simulink subsystem "Linear2Global_AV"  (R2024b)
settings: Solver=VariableStepAuto  StartTime=0.0  StopTime=10.0  RelTol=1e-3
settings Model: Creator=marti  LastModifiedBy=marti

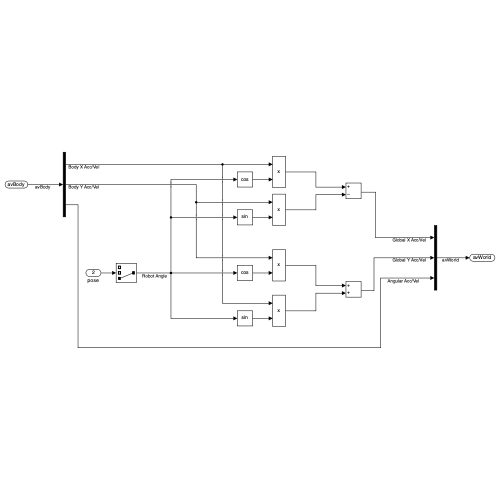
[thumbnail: Simulink's stored preview of the top-level diagram]
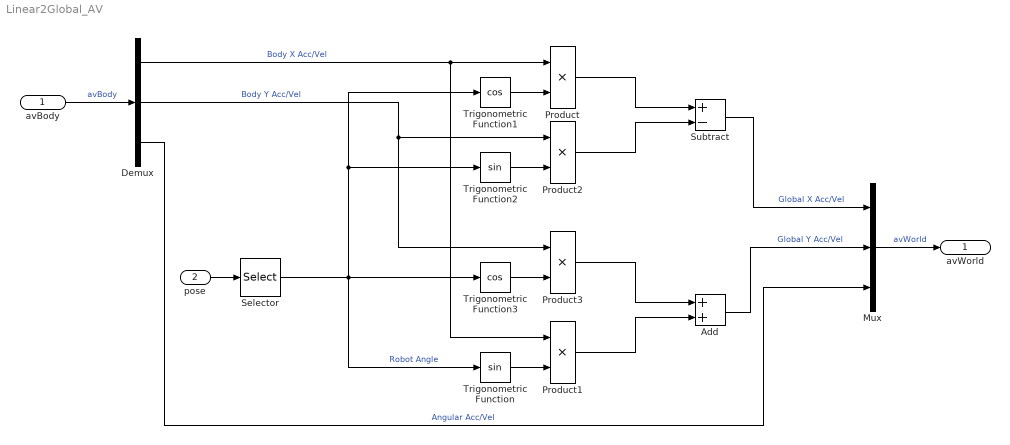
== system Linear2Global_AV ==
  avBody : Inport
  pose : Inport  Port=2
  Add : Sum
  Demux : Demux  Outputs=3
  Mux : Mux  Inputs=3
  Product{,1..3} (4 alike) : Product
  Selector : Selector  InputPortWidth=3  IndexOptions=Index vector (dialog)  Indices=3  OutputSizes=1
  Subtract : Sum  Inputs=+-
  Trigonometric Function : Trigonometry
  Trigonometric Function1 : Trigonometry  Operator=cos
  Trigonometric Function2 : Trigonometry
  Trigonometric Function3 : Trigonometry  Operator=cos
  avWorld : Outport  VectorParamsAs1DForOutWhenUnconnected=off
  wires:
  Product/1 -> Subtract/1
  Subtract/1 -> Mux/1  "Global X Acc/Vel"
  Product1/1 -> Add/2
  pose/1 -> Selector/1
  Demux/1 -> Product/1, Product1/1  "Body X Acc/Vel"
  avBody/1 -> Demux/1  "avBody"
  Trigonometric Function1/1 -> Product/2
  Selector/1 -> Trigonometric Function/1, Trigonometric Function1/1, Trigonometric Function2/1, Trigonometric Function3/1  "Robot Angle"
  Trigonometric Function3/1 -> Product3/2
  Trigonometric Function/1 -> Product1/2
  Product3/1 -> Add/1
  Add/1 -> Mux/2  "Global Y Acc/Vel"
  Trigonometric Function2/1 -> Product2/2
  Product2/1 -> Subtract/2
  Demux/2 -> Product2/1, Product3/1  "Body Y Acc/Vel"
  Mux/1 -> avWorld/1  "avWorld"
  Demux/3 -> Mux/3  "Angular Acc/Vel"
